simulink model "rtlsdr_am_envelope_demod"  (R2021a)
settings: Solver=ode45  StartTime=0.0  StopTime=60  RelTol=1e-3  EnableMultiTasking=on
PreLoadFcn:
  | %%%%%%%%%%%%%%%%%%%%%%%%%%%%%%%%%%%%%%%%%%%%%%%%%%%%%%%%%%%%%%%%%%%%%%%%%%%
  | % check to see if Simulink library folder is missing from the MATLAB path %
  | %%%%%%%%%%%%%%%%%%%%%%%%%%%%%%%%%%%%%%%%%%%%%%%%%%%%%%%%%%%%%%%%%%%%%%%%%%%
  | if isempty(strfind(path, 'rtlsdr_book_library'))
  | 
  |     % create error window
  |     fig_error = figure(...
  |         'Name', 'Error: RTL-SDR Book Library',...
  |         'Toolbar','none',...
  |         'MenuBar','none',...
  |         'NumberTitle','off',...
  |         'Resize','off',...
  |         'WindowStyle','modal');
  |     fig_error.Position(3) = 600;
  |     fig_error.Position(4) = 150;
  |     fig_axes = axes(...
  |         'Parent',fig_error,...
  |         'Position',[0,0,1,1],...
  |         'visible','off');
  |     % error message
  |     t_title = text(.05,.8,...
  |         'MISSING DIRECTORIES',...
  |         'FontSize',11.5);
  |     t_body = text(.075,.6,...
  |         [{'Simulink cannot find the  \it{<root>}\rm / \it{rtlsdr\_book\_library}\rm  folder in the \it{MATLAB Path}\rm.'},...
  |         {'Please set the MATLAB path following the instructions given in Exercise 2.4.'}],...
  |         'FontSize',10.5);
  |     % buttons
  |     btn_path = uicontrol(...
  |         'Parent',fig_error,...
  |         'String','Set Path Now',...
  |         'FontSize',10,...
  |         'Callback', 'pathtool; close(fig_error);',...
  |         'Position', [fig_error.Position(3)/2-210, 30, 200, 30]);
  |     btn_abort = uicontrol(...
  |         'Parent',fig_error,...
  |         'String','No thanks',...
  |         'FontSize',10,...
  |         'Callback', 'close(fig_error); abort=1;',...
  |         'Position', [fig_error.Position(3)/2+10, 30, 200, 30]);
  | 
  |     % pause to allow user to interact with error box
  |     uiwait(fig_error);
  | 
  |     % abort simulation
  |     try
  |         if abort==1
  |             set_param(gcs, 'SimulationCommand', 'stop');
  |         end
  |     end
  | 
  |     % if user has set path, allow diagram to be updated
  |     if ~exist('abort','var')
  |         % create error window
  |         fig_update = figure(...
  |             'Name', 'Update Diagram',...
  |             'Toolbar','none',...
  |             'MenuBar','none',...
  |             'NumberTitle','off',...
  |             'Resize','off');
  |         fig_update.Position(3) = 400;
  |         fig_update.Position(4) = 120;
  |         fig_axes = axes(...
  |             'Parent',fig_update,...
  |             'Position',[0,0,1,1],...
  |             'visible','off');
  |         % instruction message
  |         t_body = text(.075,.7,...
  |             'Once you have set the path, update the block diagram',...
  |             'FontSize',10.5);
  |         % button
  |         btn_update = uicontrol(...
  |             'Parent',fig_update,...
  |             'String','Update Block Diagram',...
  |             'FontSize',10,...
  |             'Callback', 'set_param(gcs,''SimulationCommand'',''update''); close(gcf)',...
  |             'Position', [fig_update.Position(3)/2-100, 30, 200, 30]);
  |     end
  | 
  |     % clear error components
  |     clear('fig_error','fig_update','fig_axes','t_title','t_body','btn_path','btn_abort','btn_update','abort');
  | 
  | end
  | %%%%%%%%%%%%%%%%%%%%%%%%%%%%%%%%%%%%%%%%%%%%%%%%%%%%%%%%%%%%%%%%%%%%%%%%%%%
undefined symbols (not defined in the file or in its folder): fdesignblkfcn, gcbh
libraries: rtlsdr_book_library x2, dspsnks4 x1, dspmlti4 x1, sdrrlib x1
CloseFcn:
  | closefcn_model;
Description:
  | Software, Simulation Examples and Design Exercises Licence Agreement
  | 
  | This license agreement refers to the simulation examples, design exercises and files,
  | and associated software MATLAB and Simulink resources that accompany the book:
  | 
  |      Title: Software Defined Radio using MATLAB & Simulink and the RTL-SDR
  |      Published by Strathclyde Academic Media, 2015
  |      Authored by Robert W. Stewart, Kenneth W. Barlee, Dale S.W. Atkinson,
  |      and Louise H. Crockett
  | 
  | and made available as a download from, www.desktopSDR.com or variously acquired
  | by other means such as via USB storage, cloud storage, disk or any other electronic
  | or optical or magnetic storage mechanism. These files and associated software may
  | be used subject to the terms of agreement of the conditions below:
  | 
  |     Copyright © 2015 Robert W. Stewart, Kenneth W. Barlee, Dale S.W. Atkinson,
  |     and Louise H. Crockett
  |     All rights reserved.
  | 
  | Redistribution and use in source and binary forms, with or without modification, are
  | permitted provided that the following conditions are met:
  | 
  |    1.  Redistributions of source code must retain the above copyright notice, this list of
  |         conditions and the following disclaimer.
  | 
  |    2.  Redistributions in binary form must reproduce the above copyright notice, this
  |         list of conditions and the following disclaimer in the documentation and/or other
  |         materials provided with the distribution.
  | 
  |    3.  Neither the name of the copyright holder nor the names of its contributors may
  |         be used to endorse or promote products derived from this software without
  |         specific prior written permission.
  | 
  |    4.  In all cases, the software is, and all modifications and derivatives of the
  |         software shall be, licensed to you solely for use in conjunction with The
  |         MathWorks, Inc. products and service offerings.
  | 
  | THIS SOFTWARE IS PROVIDED BY THE COPYRIGHT HOLDERS AND CONTRIBUTORS
  | "AS IS" AND ANY EXPRESS OR IMPLIED WARRANTIES, INCLUDING, BUT NOT LIMITED
  | TO, THE IMPLIED WARRANTIES OF MERCHANTABILITY AND FITNESS FOR A
  | PARTICULAR PURPOSE ARE DISCLAIMED. IN NO EVENT SHALL THE COPYRIGHT
  | HOLDER OR CONTRIBUTORS BE LIABLE FOR ANY DIRECT, INDIRECT, INCIDENTAL,
  | SPECIAL, EXEMPLARY, OR CONSEQUENTIAL DAMAGES (INCLUDING, BUT NOT
  | LIMITED TO, PROCUREMENT OF SUBSTITUTE GOODS OR SERVICES; LOSS OF USE,
  | DATA, OR PROFITS; OR BUSINESS INTERRUPTION) HOWEVER CAUSED AND ON ANY
  | THEORY OF LIABILITY, WHETHER IN CONTRACT, STRICT LIABILITY, OR TORT
  | (INCLUDING NEGLIGENCE OR OTHERWISE) ARISING IN ANY WAY OUT OF THE USE
  | OF THIS SOFTWARE, EVEN IF ADVISED OF THE POSSIBILITY OF SUCH DAMAGE.
  | 
  | 
  | Audio Tracks used in Simulations Examples and Design Exercises
  | 
  | The music and vocal files used within the Examples files and software within the book
  | were variously written, arranged, performed, recorded and produced by Garrey Rice,
  | Adam Struth, Jamie Struth, Iain Thistlethwaite and also Marshall Craigmyle who
  | collectively, and individually where appropriate, assert and retain all of their copyright,
  | performance and artistic rights. Permission to use and reproduce this music is
  | granted for all purposes associated with MATLAB and Simulink software and the
  | simulation examples and design exercises files that accompany this book. Requests to
  | use the music for any other purpose should be directed to: info@desktopSDR.com.
  | For information on music track names, full credits, and links to the musicians please
  | refer to www.desktopSDR.com/more/audio.
settings Model: SimulationMode=accelerator  Creator=desktopSDR Team  LastModifiedBy=Alex
settings SolverCC: AlgebraicLoopSolver=TrustRegion
settings DataIOCC: SaveFormat=Array  SaveOutput=off  SignalLogging=off  SaveTime=off  ReturnWorkspaceOutputs=off
settings OptimizationCC: LifeSpan=inf
settings DebuggingCC: SolverPrmCheckMsg=warning  ParameterPrecisionLossMsg=none  SFUnexpectedBacktrackingDiag=warning  SFNoUnconditionalDefaultTransitionDiag=warning  SFExecutionAtInitializationDiag=none  SFMachineParentedDataDiag=warning  ArithmeticOperatorsInVariantConditions=warning
settings HardwareCC: ProdBitPerPointer=32  ProdBitPerSizeT=32  ProdBitPerPtrDiffT=32  ProdLargestAtomicFloat=None  ProdIntDivRoundTo=Undefined  ProdEndianess=Unspecified  ProdWordSize=32  ProdHWDeviceType=32-bit Generic
settings ModelReferenceCC: PropagateSignalLabelsOutOfModel=off
settings SFSimCC: SimUseLocalCustomCode=off  CustomCodeUndefinedFunction=UseInterfaceOnly
settings RTWCC: RTWUseLocalCustomCode=off
settings CodeAppCC: StateflowObjectComments=on
settings GRTTargetCC: TargetLangStandard=C89/C90 (ANSI)
settings ConfigComp: CovMetricSettings=dw  CovSaveCumulativeToWorkspaceVar=on  CovSaveSingleToWorkspaceVar=on  CovExternalEMLEnable=off  CovSFcnEnable=off

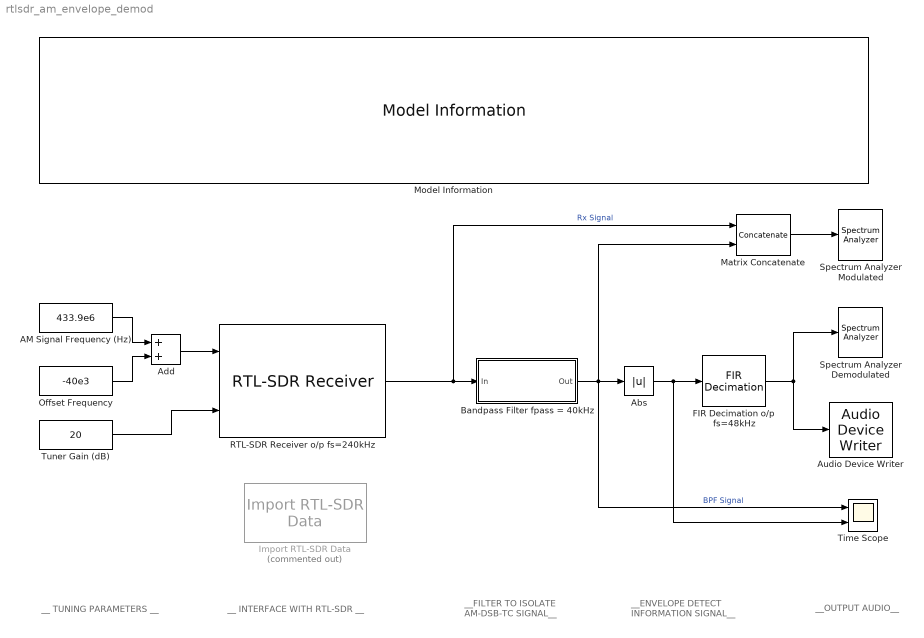
== system rtlsdr_am_envelope_demod ==
  note: __ TUNING PARAMETERS __
  note: __ INTERFACE WITH RTL-SDR __
  note: __FILTER TO ISOLATE
      | AM-DSB-TC SIGNAL__
  note: __OUTPUT AUDIO__
  note: __ENVELOPE DETECT
      | INFORMATION SIGNAL__
  AM Signal Frequency (Hz) : Constant  Value=433.9e6
  Abs : Abs
  Add : Sum
  Audio Device Writer : dspsnks4/Audio Device Writer  Driver=DirectSound  Device=Default  InheritSampleRate=on  SampleRate=44100  BitDepth=16-bit integer  BufferSize=4096  NumBuffers=10  DefaultOutputChannelMapping=on  OutputChannelMapping=1:2  OutputNumUnderrunSamples=off  DriverIdx=1  DeviceWarnFlag=''
  Bandpass Filter fpass = 40kHz : Subsystem  DialogController=fdesignblkfcn  InitFcn=fdesignblkfcn(gcbh, {'InitFcn'});  mask(Bandpass Filter){}
      mask help: Design a bandpass filter
      settings: CopyFcn=fdesignblkfcn(gcbh, {'CopyFcn'});
      mask Help: helpview(mapfilelocation('dsp'), 'dspbandpassfilter');
      mask Display: disp('Bandpass');
  FIR Decimation o/p fs=48kHz : dspmlti4/FIR Decimation  FilterSource=Dialog parameters  h=firpm(100, [0 15e3 20e3 (240e3/2)]/(240e3/2), [1 1 0 0], [1 1], 20)  D=5  filtStruct=Direct form  FilterObject=Hm_firdecim  InputProcessing=Columns as channels (frame based)  framing=Allow multirate processing  inputOffset=0  outputBufInitCond=0  roundingMode=Floor  overflowMode=off  firstCoeffDataTypeStr=Inherit: Same word length as input  firstCoeffMin=[]  firstCoeffMax=[]  firstCoeffLastDataTypeStr=Inherit: Same word length as input  outputDataTypeStr=Inherit: Same as accumulator  outputMin=[]  outputMax=[]  outputLastDataTypeStr=Inherit: Same as accumulator
  Import RTL-SDR Data : rtlsdr_book_library/Additional Tools/Import RTL-SDR Data  Commented=on  filename=rec_data/am_dsb_tc.mat  frm_size=4096  data_type=single
      settings: SourceProductName=RTL-SDR Book Library
  Matrix Concatenate : Concatenate  Mode=Multidimensional array  ConcatenateDimension=2
  Model Information : rtlsdr_book_library/Additional Tools/Model Information/Model Information
      settings: SourceProductName=RTL-SDR Book Library
  Offset Frequency : Constant  Value=-40e3
  RTL-SDR Receiver o/p fs=240kHz : sdrrlib/RTL-SDR Receiver  IPAddress=0  CenterFrequencySource=Input port  CenterFrequency=433.9e6-100e3  GainSource=Input port  Gain=40  ADCRate=240e3  FrequencyCorrection=0  LostSamplesOutputPort=off  LatencyOutputPort=off  OutputDataType=single  FrameLength=4096  EnableBurstMode=off  NumFramesInBurst=20  sobjType=sdrr.internal.SDRRTLReceiverSL  dataUDPPort=-1  ctrlUDPPort=-1  subDeviceList=nosubdev  sdrBlockType=SDRBlockTypeSLT.SDRRxBlock  requester=UNUSED_BY_SFCN  sdrExecutionMode=SDRExecutionModeSLT.ExecModeHW  BypassUserLogic=off  DecimatorSelect=DDC decimator  SourceSelect=RF data  SineAmplitude=16000  EnableInternalClock=off  BypassIQBalance=off  IFBandwidth=40e6  ADCRateSource=Dialog  IntermediateFrequency=0  DecimationFactorSource=Dialog  DecimationFactor=512  RFFrequencyIsTunable=logical(1)  SampleTime=(4096)/(240e3)  IFBandwidthSource=Dialog  SineFrequency=30000  BypassDCBlockingFilter=off  IntermediateFrequencySource=Dialog  IQBalanceCoefficients=64  SkipAllHardwareResetAndInitialization=off  EnableIQCalibrationTable=on  CacheIQCalibrationTable=off  EnableOffsetTuning=off  EnableRTLAGC=off  EnableTestMode=off  EnableTunerAGC=off  FrequencyCorrectionSource=Dialog  NumMLBuffers=128  NumUSBBuffers=16  RTLCrystalFrequency=28800000  TunerCrystalFrequency=28800000
      settings: SourceProductBaseCode=RTLSDR
  Spectrum Analyzer Demodulated : SpectrumAnalyzer
  Spectrum Analyzer Modulated : SpectrumAnalyzer
  Time Scope : Scope  NumInputPorts=2
  Tuner Gain (dB) : Constant  Value=20
  wires:
  AM Signal Frequency (Hz)/1 -> Add/1
  Offset Frequency/1 -> Add/2
  Matrix Concatenate/1 -> Spectrum Analyzer Modulated/1
  Add/1 -> RTL-SDR Receiver o/p fs=240kHz/1
  Tuner Gain (dB)/1 -> RTL-SDR Receiver o/p fs=240kHz/2
  RTL-SDR Receiver o/p fs=240kHz/1 -> Matrix Concatenate/1, Bandpass Filter fpass = 40kHz/1(In)  "Rx Signal"
  Bandpass Filter fpass = 40kHz/1(Out) -> Time Scope/1, Matrix Concatenate/2, Abs/1  "BPF Signal"
  Abs/1 -> Time Scope/2, FIR Decimation o/p fs=48kHz/1
  FIR Decimation o/p fs=48kHz/1 -> Audio Device Writer/1, Spectrum Analyzer Demodulated/1

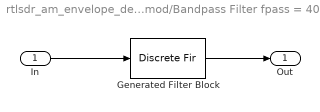
== system rtlsdr_am_envelope_demod/Bandpass Filter fpass = 40kHz ==
  In : Inport
  Generated Filter Block : DiscreteFir  Tag=BlockMethodSubSystem  Coefficients=[0.0024383680654391266 -0.0024904844872335242 0.00082961815879895701 0.00075763990941191215 -0.0029743999995476239 -0.0056956755431176696 -0.0028776958737143331 0.0020233577255912424 0.0023310659405153564 -0.00027212204672271394 0.0012989807907630405 0.0055550878283859278 0.0037368666021221309 -0.0037077560769040426 -0.0061305950204785216 -0.0015673349864665197 -0.0006454198175578085 -0.0058853330339690684 -0.0049754807192339363 0.0060584946757697815 0.012134568108140786 0.0046828751969348751 -0.0019634302976166175 0.0030583074049244036 0.0052335956968274575 -0.008152037346226635 -0.019634505516675459 -0.0095052582270241989 0.0068404420787941582 0.004788787517538428 -0.0033288481268329323 0.0090952335007954618 0.027639450416940377 0.016192021336710476 -0.015076121972225669 -0.021098373362246722 -0.0027404495183462065 -0.0071585981673002825 -0.034811306082885518 -0.02583264255396283 0.029932696481132628 0.056508405600255537 0.01934110411948356 -0.0029407606412845269 0.039788104942006325 0.047298725684134721 -0.076164128858747737 -0.20720748443321041 -0.12610208390493866 0.14072053470827206 0.29175920861567461 0.14072053470827206 -0.12610208390493866 -0.20720748443321041 -0.076164128858747737 0.047298725684134721 0.039788104942006325 -0.0029407606412845269 0.01934110411948356 0.056508405600255537 0.029932696481132628 -0.02583264255396283 -0.034811306082885518 -0.0071585981673002825 -0.0027404495183462065 -0.021098373362246722 -0.015076121972225669 0.016192021336710476 0.027639450416940377 0.0090952335007954618 -0.0033288481268329323 0.004788787517538428 0.0068404420787941582 -0.0095052582270241989 -0.019634505516675459 -0.008152037346226635 0.0052335956968274575 0.0030583074049244036 -0.0019634302976166175 0.0046828751969348751 0.012134568108140786 0.0060584946757697815 -0.0049754807192339363 -0.0058853330339690684 -0.0006454198175578085 -0.0015673349864665197 -0.0061305950204785216 -0.0037077560769040426 0.0037368666021221309 0.0055550878283859278 0.0012989807907630405 -0.00027212204672271394 0.0023310659405153564 0.0020233577255912424 -0.0028776958737143331 -0.0056956755431176696 -0.0029743999995476239 0.00075763990941191215 0.00082961815879895701 -0.0024904844872335242 0.0024383680654391266]  InputProcessing=Columns as channels (frame based)
  Out : Outport
  wires:
  Generated Filter Block/1 -> Out/1
  In/1 -> Generated Filter Block/1
